simulink model "slexClassifyAndDisplayDigitImages"  (R2021a)
settings: Solver=FixedStepDiscrete  StartTime=0.0  StopTime=600  RelTol=1e-3
libraries: dspvision x1, visiontextngfix x1, visionsinks x1
settings Model: Creator=The MathWorks, Inc.  LastModifiedBy=The MathWorks, Inc.
settings SolverCC: AlgebraicLoopSolver=TrustRegion
settings DataIOCC: ReturnWorkspaceOutputs=off
settings DebuggingCC: SFMachineParentedDataDiag=warning  ArithmeticOperatorsInVariantConditions=warning
settings SFSimCC: SimUseLocalCustomCode=off  CustomCodeUndefinedFunction=UseInterfaceOnly
settings RTWCC: RTWUseLocalCustomCode=off
settings CodeAppCC: StateflowObjectComments=on

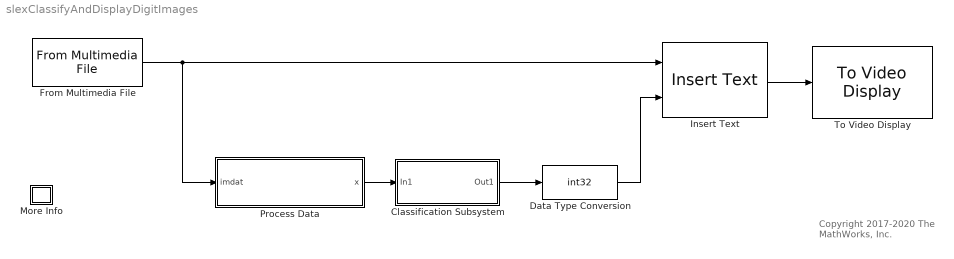
== system slexClassifyAndDisplayDigitImages ==
  note: Copyright 2017-2020 The MathWorks, Inc.
  Classification Subsystem : Subsystem  Variant=on
  Data Type Conversion : DataTypeConversion  OutDataTypeStr=int32
  From Multimedia File : dspvision/From Multimedia File  inputFilename=testImages.avi  readRange=[1 Inf]  loop=on  numPlays=inf  outputStreams=Video only  videoDataType=single  audioDataType=int16  inheritSampleTime=on  userDefinedSampleTime=1/30  noAudioOutput=off  isIntensityVideo=off  fourcc=Intensity  colorVideoFormat=One multidimensional signal  outputEOF=off  dataOrg=Column-major  audioFrameSize=1024  computeAudioFrameSize=off  outSamplingMode=Sample based
  Insert Text : visiontextngfix/Insert Text  inputType=Obsolete  theText='%d'  getTextLocFrom=Specify via dialog  textLoc=[1 1]  getTextColorFrom=Specify via dialog  textColor=[255 0 0]  getTextIntensityFrom=Specify via dialog  textIntensity=0  getTextOpacityFrom=Specify via dialog  textOpacity=1.0  dummyVar2=0  dummyVar3=0  dummyVar4=0  imagePorts=One multidimensional signal  isInputTransposed=off  fontFace=LucidaSansRegular  dummyVar1=0  blockFontSize=12  antiAliased=on
      settings: SourceProductBaseCode=VP
  More Info : Subsystem
      settings: OpenFcn=showExample('stats/SystemObjectsForClassificationAndCodeGenerationExample')
      mask Display: disp('?')
  Process Data : MATLAB Function  TreatAsAtomicUnit=on
  To Video Display : visionsinks/To Video Display  windowSizeMode=Normal  openAtMdlStart=on  fullScreen=off  videoWindowX=766  videoWindowY=438  saveWindowSize=off  videoWindowWidth=220  videoWindowHeight=149  inputColorFormat=RGB  inputType=Obsolete  imagePorts=One multidimensional signal  OutputDevice=On-screen video monitor  dataOrg=Column-major  isWindowOpen=off
  wires:
  Data Type Conversion/1 -> Insert Text/2
  Insert Text/1 -> To Video Display/1
  Process Data/1(x) -> Classification Subsystem/1(In1)
  Classification Subsystem/1(Out1) -> Data Type Conversion/1
  From Multimedia File/1 -> Process Data/1(imdat), Insert Text/1

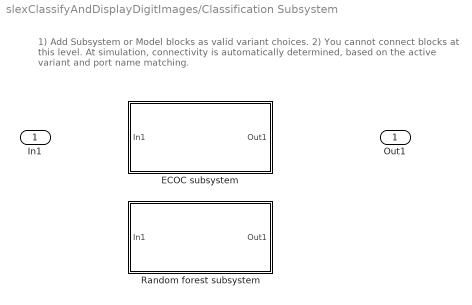
== system slexClassifyAndDisplayDigitImages/Classification Subsystem ==
  note: 1) Add Subsystem or Model blocks as valid variant choices.
      | 2) You cannot connect blocks at this level. At simulation, connectivity is automatically
      | determined, based on the active variant and port name matching.
  In1 : Inport
  ECOC subsystem : Subsystem  VariantControl=minCVLossECOC <= minCVLossRF
  Random forest subsystem : Subsystem  VariantControl=minCVLossECOC > minCVLossRF
  Out1 : Outport  VectorParamsAs1DForOutWhenUnconnected=off

== system slexClassifyAndDisplayDigitImages/More Info ==

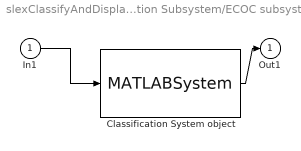
== system slexClassifyAndDisplayDigitImages/Classification Subsystem/ECOC subsystem ==
  In1 : Inport
  Classification System object : MATLABSystem  System=ECOCClassifier  SimulateUsing=Code generation
      mask Type: ECOCClassifier
      mask Display:
      | disp('ECOCClassifier');
      | port_label('input',1,'u');
      | port_label('output',1,'y');
  Out1 : Outport  VectorParamsAs1DForOutWhenUnconnected=off
  wires:
  In1/1 -> Classification System object/1
  Classification System object/1 -> Out1/1

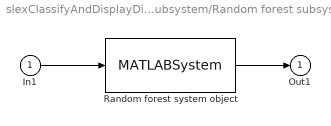
== system slexClassifyAndDisplayDigitImages/Classification Subsystem/Random forest subsystem ==
  In1 : Inport
  Random forest system object : MATLABSystem  System=RFClassifier  SimulateUsing=Code generation
      mask Type: RFClassifier
      mask Display:
      | disp('RFClassifier');
      | port_label('input',1,'u');
      | port_label('output',1,'y');
  Out1 : Outport  VectorParamsAs1DForOutWhenUnconnected=off
  wires:
  In1/1 -> Random forest system object/1
  Random forest system object/1 -> Out1/1

== matlab function slexClassifyAndDisplayDigitImages/Process Data ==
  data: imdat input; x output
function x = scalePixelIntensities(imdat)
%SCALEPIXELINTENSITIES Scales image pixel intensities
%   SCALEPIXELINTENSITIES scales the pixel intensities of the image such
%   that the result x is a row vector of values in the interval [0,1].

imdat = imdat(:)';
minimdat = min(min(imdat));
maximdat = max(max(imdat));
x = (imdat - minimdat)/(maximdat - minimdat);

end
